simulink model "part_3"  (R2025b)
settings: Solver=VariableStepAuto  StartTime=0.0  StopTime=10.0  RelTol=1e-3
libraries: dspxfrm3 x1
settings Model: Creator=Ultor  LastModifiedBy=Ultor

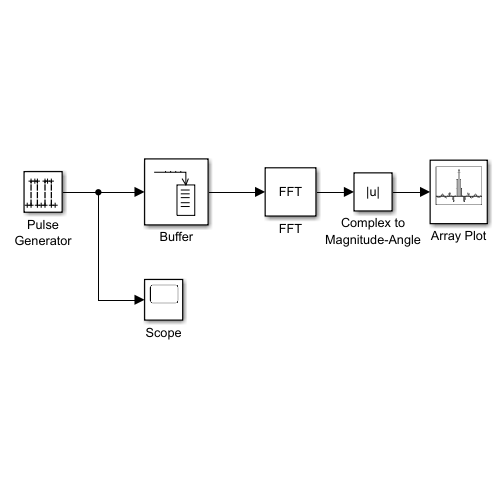
[thumbnail: Simulink's stored preview of the top-level diagram]
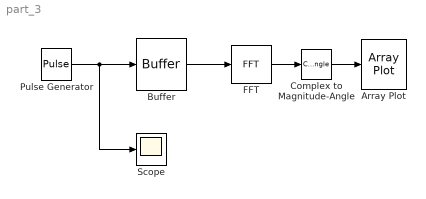
== system part_3 ==
  Array Plot : ArrayPlot  WindowPosition=[560.000000,290.000000,800.000000,500.000000,]  ScopeFrameLocation=window  YLimits=[-4 36]
  Buffer : Buffer  OutputFrames=off
  Complex to Magnitude-Angle : ComplexToMagnitudeAngle  Output=Magnitude
  FFT : dspxfrm3/FFT  FFTImplementation=Auto  CompMethod=Table lookup  TableOpt=NEW  TableOptActive=Speed  BitRevOrder=off  Normalize=off  InheritFFTLength=on  FFTLength=64  WrapInput=on  roundingMode=Ceiling  overflowMode=off  firstCoeffDataTypeStr=Inherit: Same word length as input  firstCoeffLastDataTypeStr=Inherit: Same word length as input  outputMin=[]  outputMax=[]
  Pulse Generator : DiscretePulseGenerator  Period=4  PulseWidth=2  SampleTime=1/440
  Scope : Scope
      settings: ActiveDisplayYMinimum=-0.12499999999999997  ActiveDisplayYMaximum=1.125
  wires:
  FFT/1 -> Complex to Magnitude-Angle/1
  Complex to Magnitude-Angle/1 -> Array Plot/1
  Buffer/1 -> FFT/1
  Pulse Generator/1 -> Scope/1, Buffer/1
